simulink model "parametrized_lunar_landing"  (R2016b)
settings: Solver=ode5  StartTime=0.0  StopTime=100  FixedStep=0.01  RelTol=1e-3
settings Model: Creator=Thomas  LastModifiedBy=Thomas
settings DataIOCC: SaveFormat=Array  SaveOutput=off  SaveTime=off

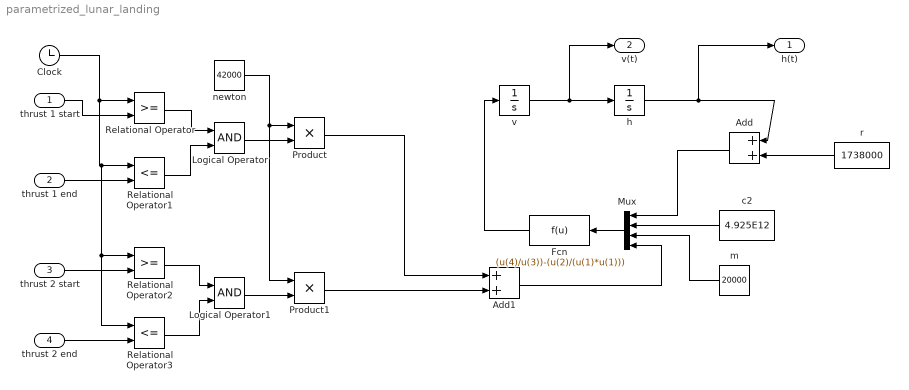
== system parametrized_lunar_landing ==
  thrust 1 start : Inport
  thrust 1 end : Inport  Port=2
  thrust 2 start : Inport  Port=3
  thrust 2 end : Inport  Port=4
  Add : Sum
  Add1 : Sum
  Clock : Clock
  Fcn : Fcn  Expr=(u(4)/u(3))-(u(2)/(u(1)*u(1)))
  Logical Operator : Logic  AllPortsSameDT=off  OutDataTypeStr=boolean
  Logical Operator1 : Logic  AllPortsSameDT=off  OutDataTypeStr=boolean
  Mux : Mux
  Product : Product
  Product1 : Product
  Relational Operator : RelationalOperator  OutDataTypeStr=boolean  RndMeth=Simplest
  Relational Operator1 : RelationalOperator  Operator=<=  OutDataTypeStr=boolean  RndMeth=Simplest
  Relational Operator2 : RelationalOperator  OutDataTypeStr=boolean  RndMeth=Simplest
  Relational Operator3 : RelationalOperator  Operator=<=  OutDataTypeStr=boolean  RndMeth=Simplest
  c2 : Constant  Value=4.925E12
  h : Integrator  InitialCondition=1000
  m : Constant  Value=20000
  newton : Constant  Value=42000
  r : Constant  Value=1738000
  v : Integrator  InitialCondition=-10
  h(t) : Outport
  v(t) : Outport  Port=2
  wires:
  v/1 -> v(t)/1, h/1
  Mux/1 -> Fcn/1
  h/1 -> h(t)/1, Add/1
  r/1 -> Add/2
  Add/1 -> Mux/1
  c2/1 -> Mux/2
  m/1 -> Mux/3
  Add1/1 -> Mux/4
  Fcn/1 -> v/1
  Clock/1 -> Relational Operator3/1, Relational Operator2/1, Relational Operator1/1, Relational Operator/1
  thrust 1 start/1 -> Relational Operator/2
  thrust 1 end/1 -> Relational Operator1/2
  Relational Operator/1 -> Logical Operator/1
  Relational Operator1/1 -> Logical Operator/2
  newton/1 -> Product/1, Product1/1
  Logical Operator/1 -> Product/2
  thrust 2 start/1 -> Relational Operator2/2
  thrust 2 end/1 -> Relational Operator3/2
  Relational Operator2/1 -> Logical Operator1/1
  Relational Operator3/1 -> Logical Operator1/2
  Logical Operator1/1 -> Product1/2
  Product/1 -> Add1/1
  Product1/1 -> Add1/2
